simulink model "test123"  (R2024b)
settings: Solver=VariableStepAuto  StartTime=0.0  StopTime=5  RelTol=1e-3
model workspace (MAT data in the model file):
  D = Simulink.Parameter
  D.Complexity = 'real'
  D.Dimensions = [0 0]
  D.DataType = 'auto'
undefined symbols (not defined in the file): Ion, Lithium
libraries: spsVoltageMeasurementLib x14, spsSeriesRLCBranchLib x12, spsCurrentMeasurementLib x10, spsMosfetLib x6, spsBatteryLib x2, slpidlib x2, spsTriangleGeneratorLib x2, spsDiodeLib x2, spsPVArrayLib x2, sps_lib x1
settings Model: Creator=pansi  LastModifiedBy=ASUS

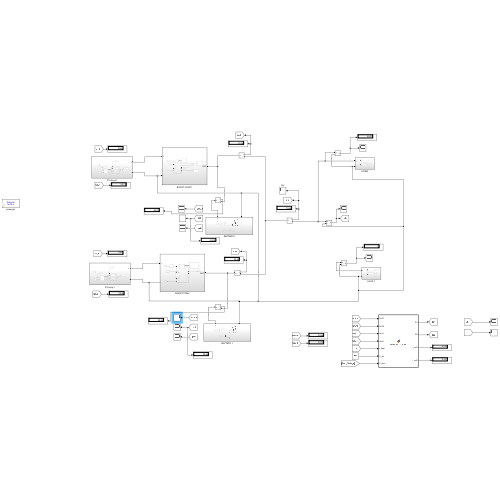
[thumbnail: Simulink's stored preview of the top-level diagram]
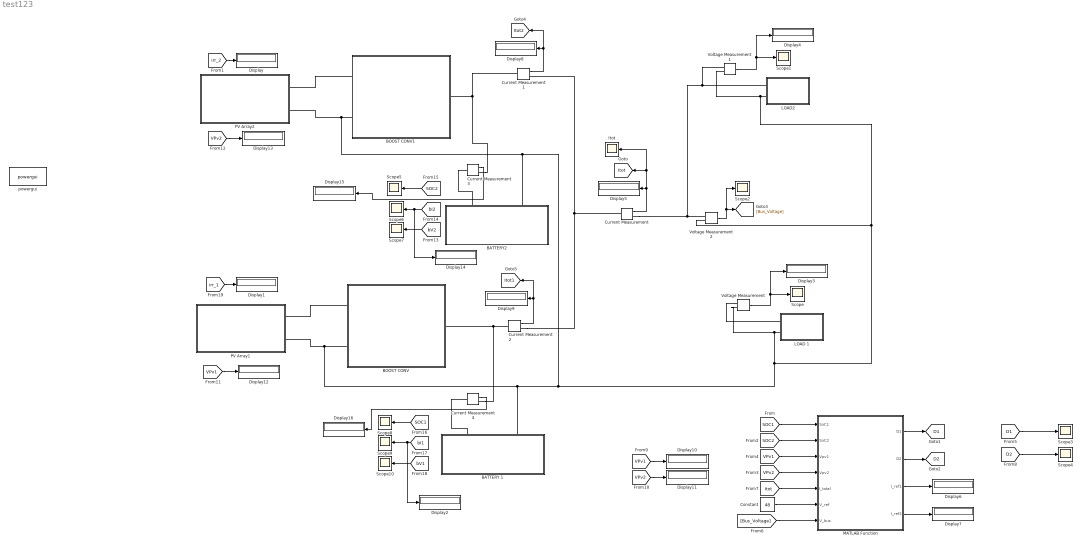
== system test123 ==
  BATTERY 1 : Subsystem
      settings: PortSchema="{\"entries\":[{\"content\":{\"sides\":[{\"content\":{},\"type\":\"ConnectorPlacement.EquallySpacedRectSide\",\"uuid\":\"5e2d450d-0339-44fd-b4b3-2e4301ef0e7a\"},{\"content\":{\"side\":\"RIGHT\"},\"type\":\"ConnectorPlacement.EquallySpacedRectSide\",\"uuid\":\"d5fab829-9fd0-4afc-851d-34441a4dac29\"},{\"content\":{\"connectorIds\":[\"LConn1\",\"LConn2\"],\"side\":\"TOP\"},\"type\":\"ConnectorPlacement.EquallySpacedRectSide\",\"uuid\":\"95d762df-4dc2-45a0-a2a5-21d0b6b4be1b\"}]},\"type\":\"ConnectorPlacement.EquallySpacedConnector\",\"uuid\":\"73cc16ff-3ada-4c0c-9ced-66d1b4be76f8\"}],\"packageUris\":[\"http://schema.mathworks.com/mf0/Connector/R2020b\"],\"version\":\"1.0\"}"
  BATTERY2 : Subsystem
      settings: PortSchema="{\"entries\":[{\"content\":{\"sides\":[{\"content\":{},\"type\":\"ConnectorPlacement.EquallySpacedRectSide\",\"uuid\":\"5e2d450d-0339-44fd-b4b3-2e4301ef0e7a\"},{\"content\":{\"side\":\"RIGHT\"},\"type\":\"ConnectorPlacement.EquallySpacedRectSide\",\"uuid\":\"d5fab829-9fd0-4afc-851d-34441a4dac29\"},{\"content\":{\"connectorIds\":[\"LConn1\",\"LConn2\"],\"side\":\"TOP\"},\"type\":\"ConnectorPlacement.EquallySpacedRectSide\",\"uuid\":\"95d762df-4dc2-45a0-a2a5-21d0b6b4be1b\"}]},\"type\":\"ConnectorPlacement.EquallySpacedConnector\",\"uuid\":\"73cc16ff-3ada-4c0c-9ced-66d1b4be76f8\"}],\"packageUris\":[\"http://schema.mathworks.com/mf0/Connector/R2020b\"],\"version\":\"1.0\"}"
  BOOST CONV : Subsystem
  BOOST CONV1 : Subsystem
  Constant : Constant  Value=48
  Current Measurement{,1..4} (5 alike) : spsCurrentMeasurementLib/Current Measurement  PhasorSimulation=off  OutputType=Complex  PSBequivalent=0
  Display{,1..16} (17 alike) : Display
  Itot : Scope
  LOAD 1 : Subsystem
  LOAD2 : Subsystem
  MATLAB Function : MATLAB Function  TreatAsAtomicUnit=on
  PV Array1 : Subsystem
  PV Array2 : Subsystem
  Scope{,1..10} (11 alike) : Scope
  Voltage Measurement : spsVoltageMeasurementLib/Voltage Measurement  PhasorSimulation=off  OutputType=Complex  PSBequivalent=0
  Voltage Measurement1 : spsVoltageMeasurementLib/Voltage Measurement  PhasorSimulation=off  OutputType=Complex  PSBequivalent=0
  Voltage Measurement2 : spsVoltageMeasurementLib/Voltage Measurement  PhasorSimulation=off  OutputType=Complex  PSBequivalent=0
  powergui : sps_lib/powergui  Priority=1  SimulationMode=Discrete  SampleTime=1e-6  frequency=60  Iterations=50  frequencyindice=0  Pbase=100e6  ErrMax=1e-4  UnitsV=kV  UnitsW=MW  buscounter=0  FunctionMessages=off  echomessages=off  EnableUseOfTLC=off  CurrentSourceSwitches=off  DisableSnubberDevices=off  DisableRonSwitches=off  DisableVfSwitches=off  DisplayEquations=off  AutomaticDiscreteSolvers=off  SolverType=Tustin/Backward Euler (TBE)  Interpol=off  ExternalGateDelay=off  methode=off  Ts=100  x0status=blocks  SPID=on  SwTol=0  HookPort=off  NonlinearTolerance=1e-4  nMaxIteration=100  ContinueOnMaxIteration=off  RestoreLinks=warning  ResistiveCurrentMeasurement=off  Frange=[0:2:500]  Ylog=off  Xlog=on  ShowGrid=off  save=off  variable=ZData  structure=0  ZoomFFT=off  StartTime=0.0  cycles=1  DisplayStyle=1  fundamental=60  FreqAxis=off  MaxFrequency=1000  frequencyindicesteady=1  RmsSteady=1  display=off
  tag scope: D1=global, D2=global, Itot1=global, Itot2=global, Itot=global
  wires:
  Voltage Measurement/1 -> Display3/1, Scope/1
  Voltage Measurement1/1 -> Scope1/1, Display4/1
  [SOC2] -> MATLAB Function/2(SoC2)
  [SOC1] -> MATLAB Function/1(SoC1)
  [VPv2] -> MATLAB Function/4(Vpv2)
  [VPv1] -> MATLAB Function/3(Vpv1)
  Constant/1 -> MATLAB Function/6(V_ref)
  Current Measurement/1 -> Itot/1, [Itot], Display5/1
  MATLAB Function/1(D1) -> [D1]
  MATLAB Function/2(D2) -> [D2]
  MATLAB Function/3(I_ref1) -> Display6/1
  MATLAB Function/4(I_ref2) -> Display7/1
  Voltage Measurement2/1 -> [Bus_Voltage], Scope2/1
  [Bus_Voltage] -> MATLAB Function/7(V_bus)
  [D1] -> Scope3/1
  Current Measurement1/1 -> Display8/1, [Itot2]
  Current Measurement2/1 -> [Itot1], Display9/1
  [D2] -> Scope4/1
  [Itot] -> MATLAB Function/5(I_total)
  [VPv1] -> Display10/1
  [VPv2] -> Display11/1
  [VPv2] -> Display13/1
  [VPv1] -> Display12/1
  [SOC2] -> Scope5/1
  [bI2] -> Display14/1, Scope6/1
  [bV2] -> Scope7/1
  [SOC1] -> Scope8/1
  [bI1] -> Display2/1, Scope9/1
  [bV1] -> Scope10/1
  [irr_2] -> Display/1
  [irr_1] -> Display1/1
  Current Measurement3/1 -> Display15/1
  Current Measurement4/1 -> Display16/1
  connections:
  BOOST CONV/LConn1 -- PV Array1/RConn1
  BOOST CONV1/LConn1 -- PV Array2/RConn1
  Current Measurement2/LConn1 -- BOOST CONV/RConn1 -- Current Measurement4/RConn1
  BOOST CONV1/LConn2 -- Voltage Measurement2/LConn2 -- Voltage Measurement1/LConn2 -- LOAD2/LConn2 -- Voltage Measurement/LConn2 -- LOAD 1/LConn2 -- BOOST CONV/LConn2 -- PV Array1/RConn2 -- BATTERY 1/LConn2 -- BATTERY2/LConn2 -- PV Array2/RConn2
  Voltage Measurement/LConn1 -- LOAD 1/LConn1
  Current Measurement1/LConn1 -- Current Measurement3/RConn1 -- BOOST CONV1/RConn1
  Current Measurement/LConn1 -- Current Measurement2/RConn1 -- Current Measurement1/RConn1
  BATTERY2/LConn1 -- Current Measurement3/LConn1
  BATTERY 1/LConn1 -- Current Measurement4/LConn1
  Voltage Measurement2/LConn1 -- Voltage Measurement1/LConn1 -- LOAD2/LConn1 -- Current Measurement/RConn1

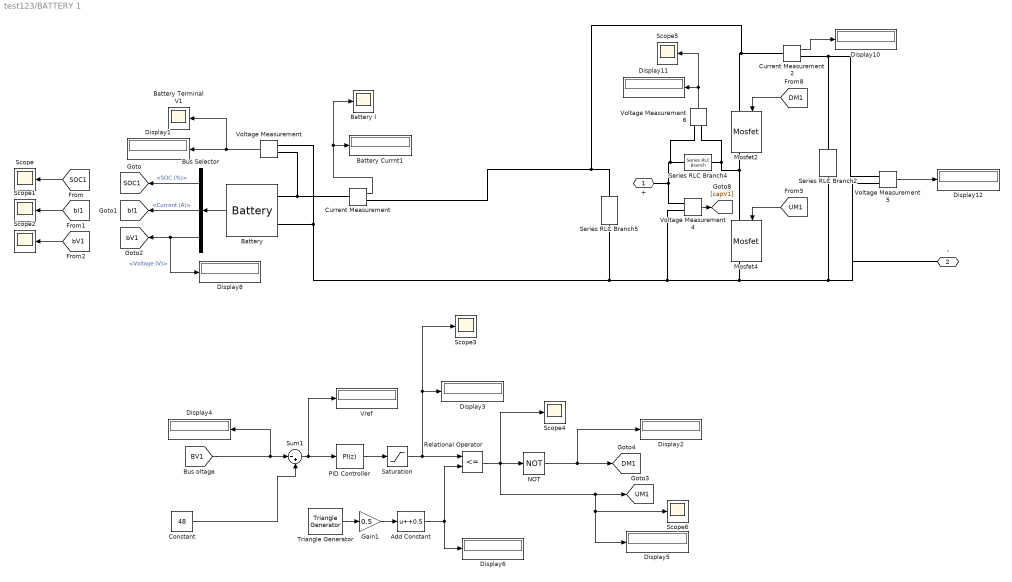
== system test123/BATTERY 1 ==
  Add Constant : Bias  Bias=+0.5  SaturateOnIntegerOverflow=off
  Battery : spsBatteryLib/Battery  BatType=Lithium-Ion  NomV=48  NomQ=100  SOC=25  Batt_Tr=1  PresetModel=off  MaxQ=111  MinV=40  FullV=54.75  Dis_rate=20  R=0.05  Normal_OP=100  expZone=[51.6,10]
  Battery Currnt1 : Display
  Battery I : Scope
  Battery Terminal V1 : Scope
  Bus Selector : BusSelector  OutputSignals=SOC (%),Current (A),Voltage (V)
  Constant : Constant  Value=48
  Current Measurement : spsCurrentMeasurementLib/Current Measurement  PhasorSimulation=off  OutputType=Complex  PSBequivalent=0
  Current Measurement2 : spsCurrentMeasurementLib/Current Measurement  PhasorSimulation=off  OutputType=Complex  PSBequivalent=0
  Display{1..6,8,10..12} (10 alike) : Display
  Gain1 : Gain  Gain=0.5
  Mosfet2 : spsMosfetLib/Mosfet  Ron=0.1  Lon=0  Rd=0.01  Vfd=0  IC=0  Rs=1e6  Cs=inf  Measurements=on
  Mosfet4 : spsMosfetLib/Mosfet  Ron=0.1  Lon=0  Rd=0.01  Vfd=0  IC=0  Rs=1e6  Cs=inf  Measurements=on
  NOT : Logic  Operator=NOT  IconShape=distinctive  AllPortsSameDT=off  OutDataTypeStr=boolean
  PID Controller : slpidlib/PID Controller  Controller=PI  Form=Parallel  TimeDomain=Discrete-time  UseExternalTs=off  SampleTime=-1  IntegratorMethod=Forward Euler  FilterMethod=Forward Euler  ControllerParametersSource=internal  P=0.5  I=100  UseKiTs=off  D=0  UseExternalDerivativeSource=off  N=100  UseFilter=on  TunerSelectOption=Transfer Function Based (PID Tuner App)  InitialConditionSource=internal  InitialConditionForIntegrator=0  InitialConditionForFilter=0  DifferentiatorICPrevScaledInput=0  ExternalReset=none  TrackingMode=off  Kt=1  LimitOutput=on  SatLimitsSource=internal  UpperSaturationLimit=1  LowerSaturationLimit=0  LinearizeAsGain=on  AntiWindupMode=none  Kb=1  LimitIntegrator=off  UpperIntegratorSaturationLimit=inf  LowerIntegratorSaturationLimit=-inf  POutMin=[]  POutMax=[]  IOutMin=[]  IOutMax=[]  DOutMin=[]  DOutMax=[]  NOutMin=[]  NOutMax=[]  SumOutMin=[]  SumOutMax=[]  SaturationOutMin=[]  SaturationOutMax=[]  PParamMin=[]  PParamMax=[]  IParamMin=[]  IParamMax=[]  DParamMin=[]  DParamMax=[]  NParamMin=[]  NParamMax=[]  KbParamMin=[]  KbParamMax=[]  KtParamMin=[]  KtParamMax=[]  KbOutMin=[]  KbOutMax=[]  KtOutMin=[]  KtOutMax=[]  IntegratorOutMin=[]  IntegratorOutMax=[]  FilterOutMin=[]  FilterOutMax=[]  SumI1OutMin=[]  SumI1OutMax=[]  SumI2OutMin=[]  SumI2OutMax=[]  SumI3OutMin=[]  SumI3OutMax=[]  SumI4OutMin=[]  SumI4OutMax=[]  SumDOutMin=[]  SumDOutMax=[]  DifferentiatorOutMin=[]  DifferentiatorOutMax=[]  FilterDiffOutCoefMin=[]  FilterDiffOutCoefMax=[]  ReciprocalOutMin=[]  ReciprocalOutMax=[]  SumDenOutMin=[]  SumDenOutMax=[]  SumNumOutMin=[]  SumNumOutMax=[]  DivideOutMin=[]  DivideOutMax=[]  UdiffTsProdOutMin=[]  UdiffTsProdOutMax=[]  NTsProdOutMin=[]  NTsProdOutMax=[]  UintegralTsProdOutMin=[]  UintegralTsProdOutMax=[]  UngainTsProdOutMin=[]  UngainTsProdOutMax=[]  ClampingZeroOutDataTypeStr=Inherit: Inherit via back propagation  ClampingZeroOutMin=[]  ClampingZeroOutMax=[]  FilterDenConstantOutDataTypeStr=Inherit: Inherit via back propagation  FilterDenConstantOutMin=[]  FilterDenConstantOutMax=[]  PCopyOutDataTypeStr=Inherit: Inherit via back propagation  PCopyOutMin=[]  PCopyOutMax=[]  NCopyOutDataTypeStr=Inherit: Inherit via back propagation  NCopyOutMin=[]  NCopyOutMax=[]  IntegratorContinuousStateAttributes=''  IntegratorStateMustResolveToSignalObject=off  IntegratorRTWStateStorageClass=Auto  FilterContinuousStateAttributes=''  FilterStateMustResolveToSignalObject=off  FilterRTWStateStorageClass=Auto  ParallelPVariant=InternalParameters  IdealPVariant=Disabled  IVariant=InternalParameters  DVariant=Disabled  IntegratorVariant=Discrete  SatVariant=Enabled  AWVariant=Passthrough  PCopyVariant=Disabled  TRVariant=Disabled  FdbkBlocksVariant=Forward  IdealPFdbkVariant=Disabled  SatFdbkVariant=Disabled  DerivativeFilterVariant=Disabled  NVariant=Disabled  NCopyVariant=Disabled_SignalSpec  FilterICVariant=Disabled  IntegratorICVariant=InternalICs  ExternalResetVariant=Disabled  TRSumVariant=Passthrough  SumFdbkVariant=Disabled  SumVariant=Sum_PI  TsampFilterVariant=InternalTs  TsampNgainVariant=Passthrough  TsampIntegralVariant=Disabled_SignalSpec  ExternalSaturationOutDataTypeStr=Inherit: Same as second input  DerivativeSourceVariant=Disabled  PreIntVariant=InternalPreInt
  Relational Operator : RelationalOperator  Operator=<=  OutDataTypeStr=boolean  RndMeth=Simplest  InputSameDT=off
  Saturation : Saturate  UpperLimit=0.9  LowerLimit=0.1
  Scope{,1..6} (7 alike) : Scope
  Series RLC Branch2 : spsSeriesRLCBranchLib/Series RLC Branch  LConnTagsString=__new0  RConnTagsString=__new0  BranchType=RC  Resistance=1  Inductance=1e-3  SetiL0=off  InitialCurrent=0  Capacitance=470e-6  Setx0=off  InitialVoltage=0  Measurements=None
  Series RLC Branch4 : spsSeriesRLCBranchLib/Series RLC Branch  LConnTagsString=__new0  RConnTagsString=__new0  BranchType=L  Resistance=1  Inductance=10e-6  SetiL0=off  InitialCurrent=0  Capacitance=1e-6  Setx0=off  InitialVoltage=0  Measurements=None
  Series RLC Branch5 : spsSeriesRLCBranchLib/Series RLC Branch  LConnTagsString=__new0  RConnTagsString=__new0  BranchType=RC  Resistance=1  Inductance=1e-3  SetiL0=off  InitialCurrent=0  Capacitance=1500e-6  Setx0=off  InitialVoltage=0  Measurements=None
  Sum1 : Sum  Inputs=|-+
  Triangle Generator : spsTriangleGeneratorLib/Triangle Generator  Freq=20000  Phase=0  Ts=1e-5
  Voltage Measurement{,4..6} (4 alike) : spsVoltageMeasurementLib/Voltage Measurement  PhasorSimulation=off  OutputType=Complex  PSBequivalent=0
  Vref : Display
  + : PMIOPort  Side=Left
  - : PMIOPort  Port=2  Side=Left
  tag scope: DM1=global, SOC1=global, UM1=global, bI1=global, bV1=global
  wires:
  Bus Selector/2 -> [bI1]  "<Current (A)>"
  Bus Selector/3 -> Display8/1, [bV1]  "<Voltage (V)>"
  Bus Selector/1 -> [SOC1]  "<SOC (%)>"
  [bI1] -> Scope1/1
  Battery/1 -> Bus Selector/1
  [SOC1] -> Scope/1
  Current Measurement/1 -> Battery I/1, Battery Currnt1/1
  [bV1] -> Scope2/1
  Voltage Measurement/1 -> Battery Terminal V1/1, Display1/1
  Gain1/1 -> Add Constant/1
  Add Constant/1 -> Display6/1, Relational Operator/2
  [BV1] -> Sum1/1, Display4/1
  Triangle Generator/1 -> Gain1/1
  Relational Operator/1 -> Scope4/1, Display5/1, Scope6/1, [UM1], NOT/1
  Sum1/1 -> Vref/1, PID Controller/1
  Saturation/1 -> Display3/1, Scope3/1, Relational Operator/1
  PID Controller/1 -> Saturation/1
  Constant/1 -> Sum1/2
  NOT/1 -> Display2/1, [DM1]
  Current Measurement2/1 -> Display10/1
  Voltage Measurement4/1 -> [capV1]
  [DM1] -> Mosfet2/1
  [UM1] -> Mosfet4/1
  Voltage Measurement6/1 -> Scope5/1, Display11/1
  Voltage Measurement5/1 -> Display12/1
  connections:
  Voltage Measurement/LConn1 -- Current Measurement/LConn1 -- Battery/LConn1
  Voltage Measurement6/LConn1 -- Series RLC Branch4/LConn1 -- +/RConn1 -- Voltage Measurement4/LConn1
  Voltage Measurement5/LConn1 -- Series RLC Branch2/LConn1 -- Current Measurement2/RConn1
  Voltage Measurement/LConn2 -- Voltage Measurement4/LConn2 -- -/RConn1 -- Voltage Measurement5/LConn2 -- Series RLC Branch2/RConn1 -- Mosfet4/RConn1 -- Series RLC Branch5/RConn1 -- Battery/LConn2
  Voltage Measurement6/LConn2 -- Series RLC Branch4/RConn1 -- Mosfet2/RConn1 -- Mosfet4/LConn1
  Series RLC Branch5/LConn1 -- Current Measurement2/LConn1 -- Mosfet2/LConn1 -- Current Measurement/RConn1

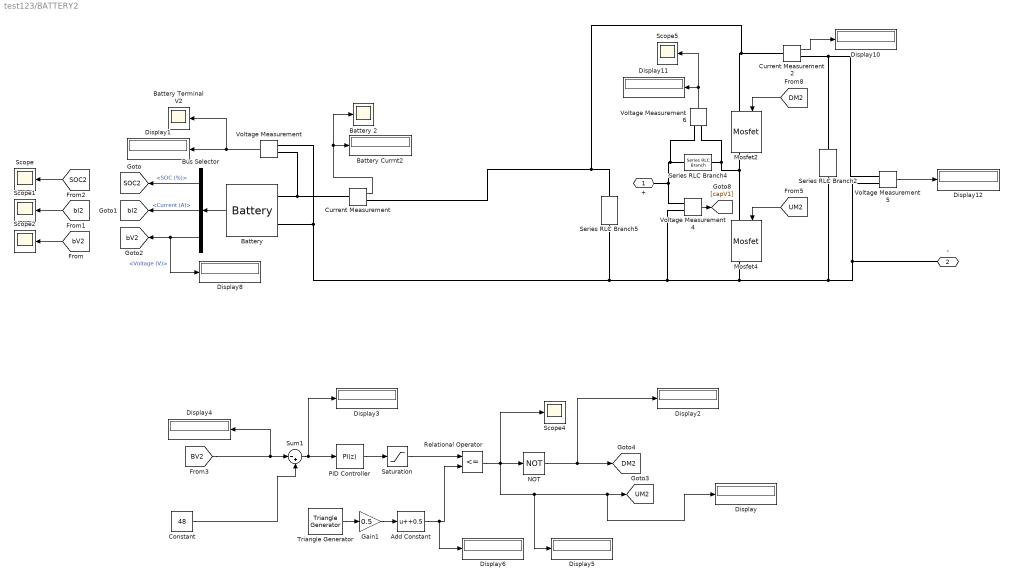
== system test123/BATTERY2 ==
  Add Constant : Bias  Bias=+0.5  SaturateOnIntegerOverflow=off
  Battery : spsBatteryLib/Battery  BatType=Lithium-Ion  NomV=48  NomQ=100  SOC=12  Batt_Tr=1  PresetModel=off  MaxQ=111  MinV=40  FullV=54.75  Dis_rate=20  R=0.05  Normal_OP=100  expZone=[51.6,10]
  Battery 2 : Scope
  Battery Currnt2 : Display
  Battery Terminal V2 : Scope
  Bus Selector : BusSelector  OutputSignals=SOC (%),Current (A),Voltage (V)
  Constant : Constant  Value=48
  Current Measurement : spsCurrentMeasurementLib/Current Measurement  PhasorSimulation=off  OutputType=Complex  PSBequivalent=0
  Current Measurement2 : spsCurrentMeasurementLib/Current Measurement  PhasorSimulation=off  OutputType=Complex  PSBequivalent=0
  Display{,1..6,8,10..12} (11 alike) : Display
  Gain1 : Gain  Gain=0.5
  Mosfet2 : spsMosfetLib/Mosfet  Ron=0.1  Lon=0  Rd=0.01  Vfd=0  IC=0  Rs=1e6  Cs=inf  Measurements=on
  Mosfet4 : spsMosfetLib/Mosfet  Ron=0.1  Lon=0  Rd=0.01  Vfd=0  IC=0  Rs=1e6  Cs=inf  Measurements=on
  NOT : Logic  Operator=NOT  IconShape=distinctive  AllPortsSameDT=off  OutDataTypeStr=boolean
  PID Controller : slpidlib/PID Controller  Controller=PI  Form=Parallel  TimeDomain=Discrete-time  UseExternalTs=off  SampleTime=-1  IntegratorMethod=Forward Euler  FilterMethod=Forward Euler  ControllerParametersSource=internal  P=0.5  I=100  UseKiTs=off  D=0  UseExternalDerivativeSource=off  N=100  UseFilter=on  TunerSelectOption=Transfer Function Based (PID Tuner App)  InitialConditionSource=internal  InitialConditionForIntegrator=0  InitialConditionForFilter=0  DifferentiatorICPrevScaledInput=0  ExternalReset=none  TrackingMode=off  Kt=1  LimitOutput=on  SatLimitsSource=internal  UpperSaturationLimit=1  LowerSaturationLimit=0  LinearizeAsGain=on  AntiWindupMode=none  Kb=1  LimitIntegrator=off  UpperIntegratorSaturationLimit=inf  LowerIntegratorSaturationLimit=-inf  POutMin=[]  POutMax=[]  IOutMin=[]  IOutMax=[]  DOutMin=[]  DOutMax=[]  NOutMin=[]  NOutMax=[]  SumOutMin=[]  SumOutMax=[]  SaturationOutMin=[]  SaturationOutMax=[]  PParamMin=[]  PParamMax=[]  IParamMin=[]  IParamMax=[]  DParamMin=[]  DParamMax=[]  NParamMin=[]  NParamMax=[]  KbParamMin=[]  KbParamMax=[]  KtParamMin=[]  KtParamMax=[]  KbOutMin=[]  KbOutMax=[]  KtOutMin=[]  KtOutMax=[]  IntegratorOutMin=[]  IntegratorOutMax=[]  FilterOutMin=[]  FilterOutMax=[]  SumI1OutMin=[]  SumI1OutMax=[]  SumI2OutMin=[]  SumI2OutMax=[]  SumI3OutMin=[]  SumI3OutMax=[]  SumI4OutMin=[]  SumI4OutMax=[]  SumDOutMin=[]  SumDOutMax=[]  DifferentiatorOutMin=[]  DifferentiatorOutMax=[]  FilterDiffOutCoefMin=[]  FilterDiffOutCoefMax=[]  ReciprocalOutMin=[]  ReciprocalOutMax=[]  SumDenOutMin=[]  SumDenOutMax=[]  SumNumOutMin=[]  SumNumOutMax=[]  DivideOutMin=[]  DivideOutMax=[]  UdiffTsProdOutMin=[]  UdiffTsProdOutMax=[]  NTsProdOutMin=[]  NTsProdOutMax=[]  UintegralTsProdOutMin=[]  UintegralTsProdOutMax=[]  UngainTsProdOutMin=[]  UngainTsProdOutMax=[]  ClampingZeroOutDataTypeStr=Inherit: Inherit via back propagation  ClampingZeroOutMin=[]  ClampingZeroOutMax=[]  FilterDenConstantOutDataTypeStr=Inherit: Inherit via back propagation  FilterDenConstantOutMin=[]  FilterDenConstantOutMax=[]  PCopyOutDataTypeStr=Inherit: Inherit via back propagation  PCopyOutMin=[]  PCopyOutMax=[]  NCopyOutDataTypeStr=Inherit: Inherit via back propagation  NCopyOutMin=[]  NCopyOutMax=[]  IntegratorContinuousStateAttributes=''  IntegratorStateMustResolveToSignalObject=off  IntegratorRTWStateStorageClass=Auto  FilterContinuousStateAttributes=''  FilterStateMustResolveToSignalObject=off  FilterRTWStateStorageClass=Auto  ParallelPVariant=InternalParameters  IdealPVariant=Disabled  IVariant=InternalParameters  DVariant=Disabled  IntegratorVariant=Discrete  SatVariant=Enabled  AWVariant=Passthrough  PCopyVariant=Disabled  TRVariant=Disabled  FdbkBlocksVariant=Forward  IdealPFdbkVariant=Disabled  SatFdbkVariant=Disabled  DerivativeFilterVariant=Disabled  NVariant=Disabled  NCopyVariant=Disabled_SignalSpec  FilterICVariant=Disabled  IntegratorICVariant=InternalICs  ExternalResetVariant=Disabled  TRSumVariant=Passthrough  SumFdbkVariant=Disabled  SumVariant=Sum_PI  TsampFilterVariant=InternalTs  TsampNgainVariant=Passthrough  TsampIntegralVariant=Disabled_SignalSpec  ExternalSaturationOutDataTypeStr=Inherit: Same as second input  DerivativeSourceVariant=Disabled  PreIntVariant=InternalPreInt
  Relational Operator : RelationalOperator  Operator=<=  OutDataTypeStr=boolean  RndMeth=Simplest  InputSameDT=off
  Saturation : Saturate  UpperLimit=0.9  LowerLimit=0.1
  Scope{,1..2,4..5} (5 alike) : Scope
  Series RLC Branch2 : spsSeriesRLCBranchLib/Series RLC Branch  LConnTagsString=__new0  RConnTagsString=__new0  BranchType=RC  Resistance=1  Inductance=1e-3  SetiL0=off  InitialCurrent=0  Capacitance=470e-6  Setx0=off  InitialVoltage=0  Measurements=None
  Series RLC Branch4 : spsSeriesRLCBranchLib/Series RLC Branch  LConnTagsString=__new0  RConnTagsString=__new0  BranchType=L  Resistance=1  Inductance=10e-6  SetiL0=off  InitialCurrent=0  Capacitance=1e-6  Setx0=off  InitialVoltage=0  Measurements=None
  Series RLC Branch5 : spsSeriesRLCBranchLib/Series RLC Branch  LConnTagsString=__new0  RConnTagsString=__new0  BranchType=RC  Resistance=1  Inductance=1e-3  SetiL0=off  InitialCurrent=0  Capacitance=1500e-6  Setx0=off  InitialVoltage=0  Measurements=None
  Sum1 : Sum  Inputs=|-+
  Triangle Generator : spsTriangleGeneratorLib/Triangle Generator  Freq=20000  Phase=0  Ts=1e-5
  Voltage Measurement{,4..6} (4 alike) : spsVoltageMeasurementLib/Voltage Measurement  PhasorSimulation=off  OutputType=Complex  PSBequivalent=0
  + : PMIOPort  Side=Left
  - : PMIOPort  Port=2  Side=Left
  tag scope: DM2=global, SOC2=global, UM2=global, bI2=global, bV2=global
  wires:
  Voltage Measurement5/1 -> Display12/1
  Voltage Measurement6/1 -> Display11/1, Scope5/1
  [UM2] -> Mosfet4/1
  [DM2] -> Mosfet2/1
  Voltage Measurement4/1 -> [capV1]
  Current Measurement2/1 -> Display10/1
  NOT/1 -> [DM2], Display2/1
  Constant/1 -> Sum1/2
  PID Controller/1 -> Saturation/1
  Saturation/1 -> Relational Operator/1
  Sum1/1 -> PID Controller/1, Display3/1
  Relational Operator/1 -> NOT/1, [UM2], Display/1, Display5/1, Scope4/1
  Triangle Generator/1 -> Gain1/1
  [BV2] -> Display4/1, Sum1/1
  Add Constant/1 -> Relational Operator/2, Display6/1
  Gain1/1 -> Add Constant/1
  Voltage Measurement/1 -> Display1/1, Battery Terminal V2/1
  [bV2] -> Scope2/1
  Current Measurement/1 -> Battery Currnt2/1, Battery 2/1
  [SOC2] -> Scope/1
  Battery/1 -> Bus Selector/1
  [bI2] -> Scope1/1
  Bus Selector/1 -> [SOC2]  "<SOC (%)>"
  Bus Selector/3 -> [bV2], Display8/1  "<Voltage (V)>"
  Bus Selector/2 -> [bI2]  "<Current (A)>"
  connections:
  Current Measurement/RConn1 -- Mosfet2/LConn1 -- Current Measurement2/LConn1 -- Series RLC Branch5/LConn1
  Mosfet4/LConn1 -- Mosfet2/RConn1 -- Series RLC Branch4/RConn1 -- Voltage Measurement6/LConn2
  Battery/LConn2 -- Series RLC Branch5/RConn1 -- Mosfet4/RConn1 -- Series RLC Branch2/RConn1 -- Voltage Measurement5/LConn2 -- -/RConn1 -- Voltage Measurement4/LConn2 -- Voltage Measurement/LConn2
  Current Measurement2/RConn1 -- Series RLC Branch2/LConn1 -- Voltage Measurement5/LConn1
  Voltage Measurement4/LConn1 -- +/RConn1 -- Series RLC Branch4/LConn1 -- Voltage Measurement6/LConn1
  Battery/LConn1 -- Current Measurement/LConn1 -- Voltage Measurement/LConn1

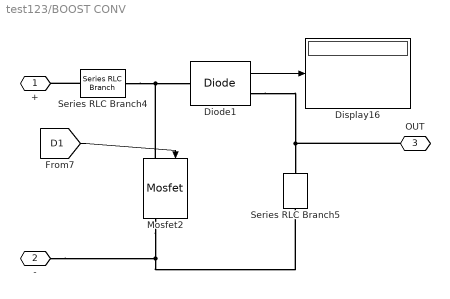
== system test123/BOOST CONV ==
  Diode1 : spsDiodeLib/Diode  Ron=0.001  Lon=0  Vf=0.8  IC=0  UseSnubber=0  Rs=500  Cs=250e-9  Measurements=on
  Display16 : Display
  Mosfet2 : spsMosfetLib/Mosfet  Ron=0.001  Lon=0  Rd=0.01  Vfd=0.8  IC=0  Rs=1e4  Cs=inf  Measurements=on
  Series RLC Branch4 : spsSeriesRLCBranchLib/Series RLC Branch  LConnTagsString=__new0  RConnTagsString=__new0  BranchType=L  Resistance=1  Inductance=100e-6  SetiL0=off  InitialCurrent=0  Capacitance=1e-6  Setx0=off  InitialVoltage=0  Measurements=None
  Series RLC Branch5 : spsSeriesRLCBranchLib/Series RLC Branch  LConnTagsString=__new0  RConnTagsString=__new0  BranchType=RC  Resistance=0.01  Inductance=1e-3  SetiL0=off  InitialCurrent=0  Capacitance=2000e-6  Setx0=off  InitialVoltage=0  Measurements=None
  + : PMIOPort  Side=Left
  - : PMIOPort  Port=2  Side=Left
  OUT : PMIOPort  Port=3  Side=Right
  wires:
  Diode1/1 -> Display16/1
  [D1] -> Mosfet2/1
  connections:
  Series RLC Branch4/RConn1 -- Diode1/LConn1 -- Mosfet2/LConn1
  Diode1/RConn1 -- Series RLC Branch5/LConn1 -- OUT/RConn1
  Series RLC Branch4/LConn1 -- +/RConn1
  Mosfet2/RConn1 -- -/RConn1 -- Series RLC Branch5/RConn1

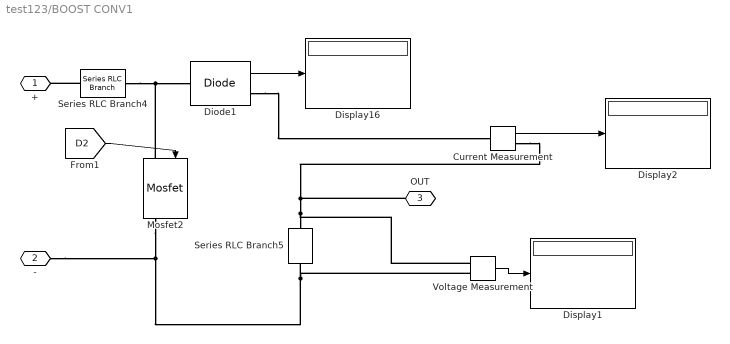
== system test123/BOOST CONV1 ==
  Current Measurement : spsCurrentMeasurementLib/Current Measurement  PhasorSimulation=off  OutputType=Complex  PSBequivalent=0
  Diode1 : spsDiodeLib/Diode  Ron=0.001  Lon=0  Vf=0.8  IC=0  UseSnubber=0  Rs=500  Cs=250e-9  Measurements=on
  Display1 : Display
  Display16 : Display
  Display2 : Display
  Mosfet2 : spsMosfetLib/Mosfet  Ron=0.001  Lon=0  Rd=0.01  Vfd=0.8  IC=0  Rs=1e4  Cs=inf  Measurements=on
  Series RLC Branch4 : spsSeriesRLCBranchLib/Series RLC Branch  LConnTagsString=__new0  RConnTagsString=__new0  BranchType=L  Resistance=1  Inductance=0.001  SetiL0=off  InitialCurrent=0  Capacitance=1e-6  Setx0=off  InitialVoltage=0  Measurements=None
  Series RLC Branch5 : spsSeriesRLCBranchLib/Series RLC Branch  LConnTagsString=__new0  RConnTagsString=__new0  BranchType=RC  Resistance=0.01  Inductance=1e-3  SetiL0=off  InitialCurrent=0  Capacitance=470e-6  Setx0=off  InitialVoltage=0  Measurements=None
  Voltage Measurement : spsVoltageMeasurementLib/Voltage Measurement  PhasorSimulation=off  OutputType=Complex  PSBequivalent=0
  + : PMIOPort  Side=Left
  - : PMIOPort  Port=2  Side=Left
  OUT : PMIOPort  Port=3  Side=Right
  wires:
  Diode1/1 -> Display16/1
  [D2] -> Mosfet2/1
  Voltage Measurement/1 -> Display1/1
  Current Measurement/1 -> Display2/1
  connections:
  -/RConn1 -- Mosfet2/RConn1 -- Voltage Measurement/LConn2 -- Series RLC Branch5/RConn1
  Series RLC Branch4/LConn1 -- +/RConn1
  OUT/RConn1 -- Current Measurement/RConn1 -- Voltage Measurement/LConn1 -- Series RLC Branch5/LConn1
  Mosfet2/LConn1 -- Diode1/LConn1 -- Series RLC Branch4/RConn1
  Diode1/RConn1 -- Current Measurement/LConn1

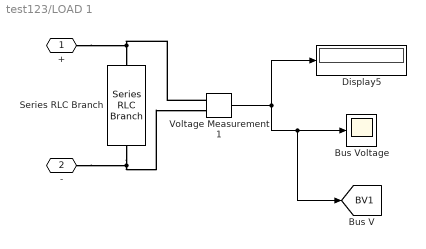
== system test123/LOAD 1 ==
  Bus Voltage : Scope
  Display5 : Display
  Series RLC Branch : spsSeriesRLCBranchLib/Series RLC Branch  LConnTagsString=__new0  RConnTagsString=__new0  BranchType=R  Resistance=4.6  Inductance=1e-3  SetiL0=off  InitialCurrent=0  Capacitance=1e-6  Setx0=off  InitialVoltage=0  Measurements=None
  Voltage Measurement1 : spsVoltageMeasurementLib/Voltage Measurement  PhasorSimulation=off  OutputType=Complex  PSBequivalent=0
  + : PMIOPort  Side=Left
  - : PMIOPort  Port=2  Side=Left
  tag scope: BV1=global
  wires:
  Voltage Measurement1/1 -> Display5/1, [BV1], Bus Voltage/1
  connections:
  Voltage Measurement1/LConn1 -- +/RConn1 -- Series RLC Branch/LConn1
  Series RLC Branch/RConn1 -- -/RConn1 -- Voltage Measurement1/LConn2

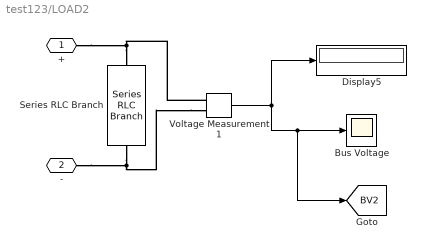
== system test123/LOAD2 ==
  Bus Voltage : Scope
  Display5 : Display
  Series RLC Branch : spsSeriesRLCBranchLib/Series RLC Branch  LConnTagsString=__new0  RConnTagsString=__new0  BranchType=R  Resistance=4.6  Inductance=1e-3  SetiL0=off  InitialCurrent=0  Capacitance=1e-6  Setx0=off  InitialVoltage=0  Measurements=None
  Voltage Measurement1 : spsVoltageMeasurementLib/Voltage Measurement  PhasorSimulation=off  OutputType=Complex  PSBequivalent=0
  + : PMIOPort  Side=Left
  - : PMIOPort  Port=2  Side=Left
  tag scope: BV2=global
  wires:
  Voltage Measurement1/1 -> [BV2], Bus Voltage/1, Display5/1
  connections:
  Voltage Measurement1/LConn2 -- -/RConn1 -- Series RLC Branch/RConn1
  Series RLC Branch/LConn1 -- +/RConn1 -- Voltage Measurement1/LConn1

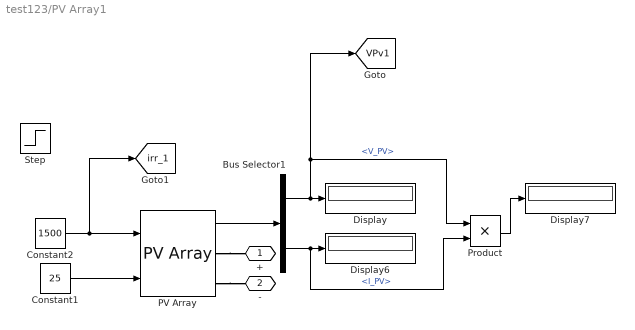
== system test123/PV Array1 ==
  Bus Selector1 : BusSelector  OutputSignals=V_PV,I_PV
  Constant1 : Constant  Value=25
  Constant2 : Constant  Value=1500
  Display : Display
  Display6 : Display
  Display7 : Display
  PV Array : spsPVArrayLib/PV Array  Npar=5  Nser=1  PlotType=array @ 1000 W/m2 & specified temperatures  S_vec="[ 1000  500  100 ]"  Temp_C_vec="[ 45 25  ]"  ModuleName=User-defined  PlotWhenSelected=off  Pm=200.143  Ncell=60  Voc=32.9  Isc=8.21  Vm=26.3  Im=7.61  beta_Voc_pc=-0.123  alpha_Isc_pc=0.0032  beta_Voc=-0.040467  alpha_Isc=0.00026272  IL=8.2568  I0=9.0626e-16  nI=0.58154  Rsh=84.0292  Rs=0.47867  RobustModel=off  RobustCellTemperature=313.3991  BAL=off  Tc=1e-6  Tfilter=5e-5
  Product : Product
  Step : Step  Before=500  After=1500  SampleTime=0
  + : PMIOPort  Side=Right
  - : PMIOPort  Port=2  Side=Right
  tag scope: VPv1=global, irr_1=global
  wires:
  Bus Selector1/2 -> Product/2, Display6/1  "<I_PV>"
  Product/1 -> Display7/1
  PV Array/1 -> Bus Selector1/1
  Constant1/1 -> PV Array/2
  Bus Selector1/1 -> [VPv1], Product/1, Display/1  "<V_PV>"
  Constant2/1 -> [irr_1], PV Array/1
  connections:
  PV Array/RConn1 -- +/RConn1
  PV Array/RConn2 -- -/RConn1

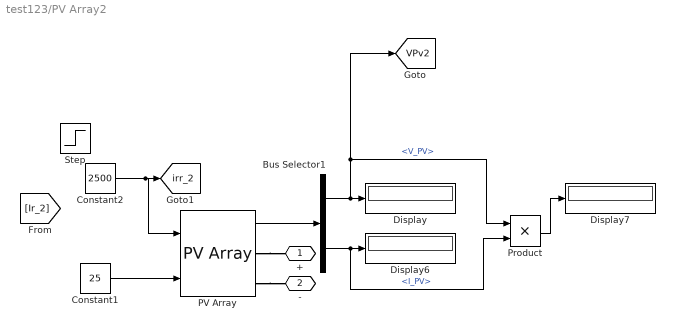
== system test123/PV Array2 ==
  Bus Selector1 : BusSelector  OutputSignals=V_PV,I_PV
  Constant1 : Constant  Value=25
  Constant2 : Constant  Value=2500
  Display : Display
  Display6 : Display
  Display7 : Display
  PV Array : spsPVArrayLib/PV Array  Npar=10  Nser=1  PlotType=array @ 1000 W/m2 & specified temperatures  S_vec="[ 1000  500  100 ]"  Temp_C_vec="[ 45 25  ]"  ModuleName=User-defined  PlotWhenSelected=off  Pm=200.143  Ncell=60  Voc=32.9  Isc=8.21  Vm=26.3  Im=7.61  beta_Voc_pc=-0.123  alpha_Isc_pc=0.0032  beta_Voc=-0.040467  alpha_Isc=0.00026272  IL=8.2568  I0=9.0626e-16  nI=0.58154  Rsh=84.0292  Rs=0.47867  RobustModel=off  RobustCellTemperature=313.3991  BAL=off  Tc=1e-6  Tfilter=5e-5
  Product : Product
  Step : Step  Before=500  After=1500  SampleTime=0
  + : PMIOPort  Side=Right
  - : PMIOPort  Port=2  Side=Right
  tag scope: VPv2=global, irr_2=global
  wires:
  Bus Selector1/1 -> Display/1, Product/1, [VPv2]  "<V_PV>"
  Constant1/1 -> PV Array/2
  PV Array/1 -> Bus Selector1/1
  Product/1 -> Display7/1
  Bus Selector1/2 -> Display6/1, Product/2  "<I_PV>"
  Constant2/1 -> [irr_2], PV Array/1
  connections:
  PV Array/RConn2 -- -/RConn1
  PV Array/RConn1 -- +/RConn1

== matlab function test123/MATLAB Function ==
  data: SoC1 input; D1 output; SoC2 input; Vpv1 input; Vpv2 input; I_total input; V_ref input; V_bus input; D2 output; I_ref1 output; I_ref2 output
function [D1, D2, I_ref1, I_ref2] = adaptive_soc_pv(...
    SoC1, SoC2, Vpv1, Vpv2, I_total, V_ref, V_bus)

%% ── INITIALIZE
D1     = 0;
D2     = 0;
I_ref1 = 0;
I_ref2 = 0;

%% ── DEFINE SoC LIMITS
SOC_FULL         = 95;  % above this → stop charging
SOC_HIGH         = 80;  % above this → reduce charge current
SOC_NORMAL_HIGH  = 60;  % normal upper band
SOC_NORMAL_LOW   = 40;  % normal lower band
SOC_LOW          = 20;  % below this → priority charge
SOC_CRITICAL     = 10;  % below this → stop discharging

%% ── VOLTAGE ERROR
e  = V_ref - V_bus;
Kp = 0.5 + 0.3 * abs(e);

%% ── PV VOLTAGE WEIGHT (60%)
Vpv_sum = Vpv1 + Vpv2 + 1e-6;
w_pv1   = 0.6 * (Vpv1 / Vpv_sum);
w_pv2   = 0.6 * (Vpv2 / Vpv_sum);

%% ── SoC DEFICIT WEIGHT (40%)
d1    = max(100 - SoC1, 0);
d2    = max(100 - SoC2, 0);
d_sum = d1 + d2 + 1e-6;
w_soc1 = 0.4 * (d1 / d_sum);
w_soc2 = 0.4 * (d2 / d_sum);

%% ── COMBINED WEIGHT
W1    = w_pv1 + w_soc1;
W2    = w_pv2 + w_soc2;
W_sum = W1 + W2 + 1e-6;

%% ── DUTY CYCLE
D_base = min(max(Kp * abs(e), 0.3), 0.95);
D1     = min(max(D_base * (W1/W_sum), 0.3), 0.95);
D2     = min(max(D_base * (W2/W_sum), 0.3), 0.95);

%% ══════════════════════════════════════════
%% BATTERY 1 — CHARGE or DISCHARGE decision
%% ══════════════════════════════════════════

if SoC1 >= SOC_FULL
    %% BATTERY 1 FULL — stop charging
    %% switch to discharge mode → supply load
    I_ref1 = -abs(I_total) * 0.3;  % discharge at 30% rate
    D1     = 0;                      % boost not needed

elseif SoC1 >= SOC_HIGH
    %% BATTERY 1 HIGH SoC (80–95%)
    %% charge slowly — nearly full
    I_ref1 = abs(I_total) * (W1/W_sum) * 0.3;  % only 30% rate

elseif SoC1 >= SOC_NORMAL_LOW
    %% BATTERY 1 NORMAL SoC (40–80%)
    %% charge proportionally — normal operation
    I_ref1 = abs(I_total) * (W1/W_sum);

elseif SoC1 >= SOC_LOW
    %% BATTERY 1 LOW SoC (20–40%)
    %% charge with HIGH current — priority
    I_ref1 = abs(I_total) * (W1/W_sum) * 1.2;  % 20% boost

elseif SoC1 >= SOC_CRITICAL
    %% BATTERY 1 CRITICAL (10–20%)
    %% emergency charge — maximum priority
    I_ref1 = abs(I_total) * 0.8;  % 80% of all current
    D1     = min(D_base * 1.2, 0.95);  % push harder

else
    %% BATTERY 1 EMPTY (below 10%)
    %% STOP discharging — protect battery
    I_ref1 = abs(I_total) * 0.9;  % maximum emergency charge
    D1     = 0.95;                  % maximum duty
end

%% ══════════════════════════════════════════
%% BATTERY 2 — CHARGE or DISCHARGE decision
%% ══════════════════════════════════════════

if SoC2 >= SOC_FULL
    %% BATTERY 2 FULL — stop charging
    %% switch to discharge → supply load
    I_ref2 = -abs(I_total) * 0.3;  % discharge at 30% rate
    D2     = 0;

elseif SoC2 >= SOC_HIGH
    %% BATTERY 2 HIGH SoC (80–95%)
    %% charge slowly
    I_ref2 = abs(I_total) * (W2/W_sum) * 0.3;

elseif SoC2 >= SOC_NORMAL_LOW
    %% BATTERY 2 NORMAL SoC (40–80%)
    %% proportional charge
    I_ref2 = abs(I_total) * (W2/W_sum);

elseif SoC2 >= SOC_LOW
    %% BATTERY 2 LOW SoC (20–40%)
    %% priority charge
    I_ref2 = abs(I_total) * (W2/W_sum) * 1.2;

elseif SoC2 >= SOC_CRITICAL
    %% BATTERY 2 CRITICAL (10–20%)
    %% emergency charge
    I_ref2 = abs(I_total) * 0.8;
    D2     = min(D_base * 1.2, 0.95);

else
    %% BATTERY 2 EMPTY (below 10%)
    %% maximum emergency charge
    I_ref2 = abs(I_total) * 0.9;
    D2     = 0.95;
end

end
